simulink model "Cascaded_LQR"  (R2021a)
settings: Solver=VariableStepAuto  StartTime=0.0  StopTime=inf  RelTol=1e-3
values from neighbouring files (symbols this model uses):
  dragCoeffMov = 0.01    [param_set.m]
  g = 9.8    [param_set.m]
  m = 1.5    [param_set.m]
  set_points = [1 0 hover_height 0 0 0 0 0 0 0 0 0]'    [linearize_lqr.m]    (also in param_set.m)
  u_eq = [T_eq 0 0 0]    [linearize_lqr.m]    (also in param_set.m = [-m*g 0 0 0])
  windVel = [0 0 0]'    [param_set.m]
undefined symbols (not defined in the file or in its folder): lqr_K
libraries: shared6dof x1, sharedtransform x1, uavutilslib x1
settings Model: Creator=willwu  LastModifiedBy=willwu

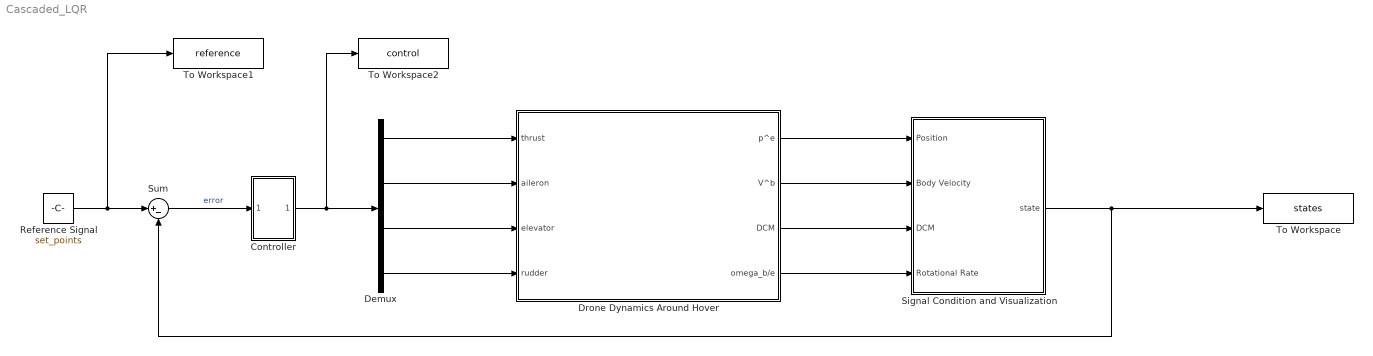
== system Cascaded_LQR ==
  Controller : Subsystem
  Demux : Demux
  Drone Dynamics Around Hover : Subsystem
  Reference Signal : Constant  Value=set_points
  Signal Condition and Visualization : Subsystem
  Sum : Sum  Inputs=|+-
  To Workspace : ToWorkspace  VariableName=states  SaveFormat=Structure With Time  SampleTime=-1
  To Workspace1 : ToWorkspace  VariableName=reference  SaveFormat=Structure With Time  SampleTime=-1
  To Workspace2 : ToWorkspace  VariableName=control  SaveFormat=Structure With Time  SampleTime=-1
  wires:
  Demux/1 -> Drone Dynamics Around Hover/1(thrust)
  Demux/2 -> Drone Dynamics Around Hover/2(aileron)
  Demux/3 -> Drone Dynamics Around Hover/3(elevator)
  Demux/4 -> Drone Dynamics Around Hover/4(rudder)
  Reference Signal/1 -> To Workspace1/1, Sum/1
  Sum/1 -> Controller/1(In1)  "error"
  Controller/1(Out1) -> Demux/1, To Workspace2/1
  Signal Condition and Visualization/1(state) -> Sum/2, To Workspace/1
  Drone Dynamics Around Hover/1(p^e) -> Signal Condition and Visualization/1(Position)
  Drone Dynamics Around Hover/2(V^b) -> Signal Condition and Visualization/2(Body Velocity)
  Drone Dynamics Around Hover/3(DCM) -> Signal Condition and Visualization/3(DCM)
  Drone Dynamics Around Hover/4(omega_b/e) -> Signal Condition and Visualization/4(Rotational Rate)

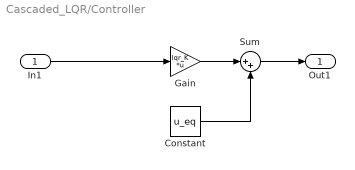
== system Cascaded_LQR/Controller ==
  In1 : Inport
  Constant : Constant  Value=u_eq
  Gain : Gain  Gain=lqr_K  Multiplication=Matrix(K*u)
  Sum : Sum  Inputs=|++
  Out1 : Outport
  wires:
  In1/1 -> Gain/1
  Gain/1 -> Sum/1
  Sum/1 -> Out1/1
  Constant/1 -> Sum/2

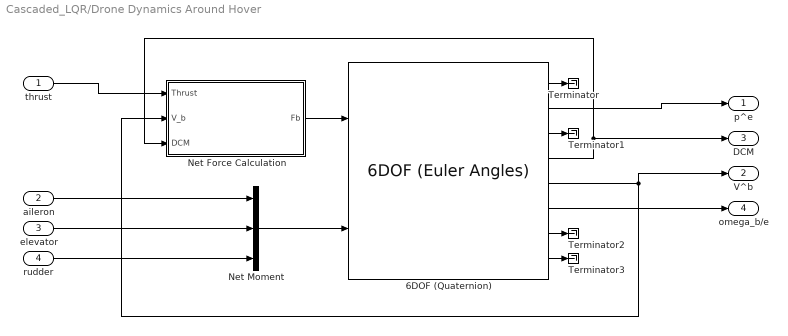
== system Cascaded_LQR/Drone Dynamics Around Hover ==
  thrust : Inport
  aileron : Inport  Port=2
  elevator : Inport  Port=3
  rudder : Inport  Port=4
  6DOF (Quaternion) : shared6dof/6DOF (Euler Angles)  units=Metric (MKS)  mtype=Fixed  rep=Quaternion  xme_0=[0 0 0]  Vm_0=[0 0 0]  eul_0=[0 0 0]  pm_0=[0 0 0]  mass_0=m  mass_e=0.5  mass_f=2.0  inertia=J  inertia_e=eye(3)  inertia_f=2*eye(3)  k_quat=1.0  vre_flag=on  abi_flag=off  aMode=0  xme_statename=''  Vm_statename=''  eul_statename=''  quat_statename=''  pm_statename=''  mass_statename=''
      settings: SourceProductBaseCode=AE,PW,DR,MT,UV,VE
  Net Force Calculation : Subsystem
  Net Moment : Mux  Inputs=3
  Terminator{,1..3} (4 alike) : Terminator
  p^e : Outport
  V^b : Outport  Port=2
  DCM : Outport  Port=3
  omega_b/e : Outport  Port=4
  wires:
  aileron/1 -> Net Moment/1
  rudder/1 -> Net Moment/3
  Net Moment/1 -> 6DOF (Quaternion)/2
  6DOF (Quaternion)/5 -> V^b/1, Net Force Calculation/2(V_b)
  6DOF (Quaternion)/6 -> omega_b/e/1
  6DOF (Quaternion)/4 -> DCM/1, Net Force Calculation/3(DCM)
  6DOF (Quaternion)/2 -> p^e/1
  thrust/1 -> Net Force Calculation/1(Thrust)
  Net Force Calculation/1(Fb) -> 6DOF (Quaternion)/1
  elevator/1 -> Net Moment/2
  6DOF (Quaternion)/1 -> Terminator/1
  6DOF (Quaternion)/3 -> Terminator1/1
  6DOF (Quaternion)/7 -> Terminator2/1
  6DOF (Quaternion)/8 -> Terminator3/1

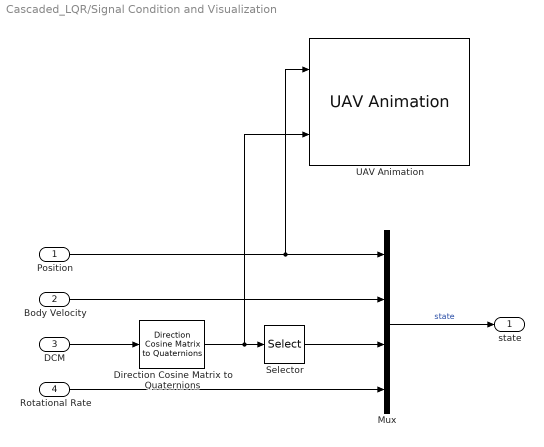
== system Cascaded_LQR/Signal Condition and Visualization ==
  Position : Inport
  Body Velocity : Inport  Port=2
  DCM : Inport  Port=3
  Rotational Rate : Inport  Port=4
  Direction Cosine Matrix to Quaternions : sharedtransform/Direction Cosine Matrix  to Quaternions  aMode=0  action=None  tolerance=eps(2)
      settings: SourceProductBaseCode=AE,PW,DR,MT,UV,VE
  Mux : Mux
  Selector : Selector  InputPortWidth=4  IndexOptions=Index vector (dialog)  Indices=[2 3 4]  OutputSizes=1
  UAV Animation : uavutilslib/UAV Animation  UAVType=Multirotor  UAVSize=1  InertialZDirection=Down  SampleTime=-1
      settings: SourceProductBaseCode=UV
  state : Outport
  wires:
  Selector/1 -> Mux/3
  Position/1 -> Mux/1, UAV Animation/1
  Body Velocity/1 -> Mux/2
  Rotational Rate/1 -> Mux/4
  Mux/1 -> state/1  "state"
  DCM/1 -> Direction Cosine Matrix to Quaternions/1
  Direction Cosine Matrix to Quaternions/1 -> Selector/1, UAV Animation/2

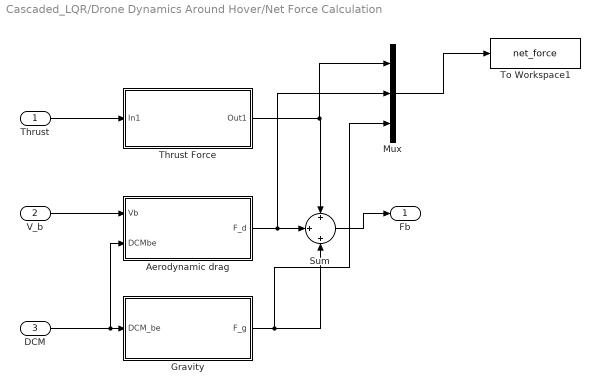
== system Cascaded_LQR/Drone Dynamics Around Hover/Net Force Calculation ==
  Thrust : Inport
  V_b : Inport  Port=2
  DCM : Inport  Port=3
  Aerodynamic drag : Subsystem
  Gravity : Subsystem
  Mux : Mux  Inputs=3
  Sum : Sum  Inputs=+|+|+
  Thrust Force : Subsystem
  To Workspace1 : ToWorkspace  VariableName=net_force  SaveFormat=Structure With Time  SampleTime=-1
  Fb : Outport
  wires:
  DCM/1 -> Aerodynamic drag/2(DCMbe), Gravity/1(DCM_be)
  Gravity/1(F_g) -> Mux/3, Sum/3
  Sum/1 -> Fb/1
  Thrust/1 -> Thrust Force/1(In1)
  Thrust Force/1(Out1) -> Mux/1, Sum/1
  V_b/1 -> Aerodynamic drag/1(Vb)
  Aerodynamic drag/1(F_d) -> Mux/2, Sum/2
  Mux/1 -> To Workspace1/1

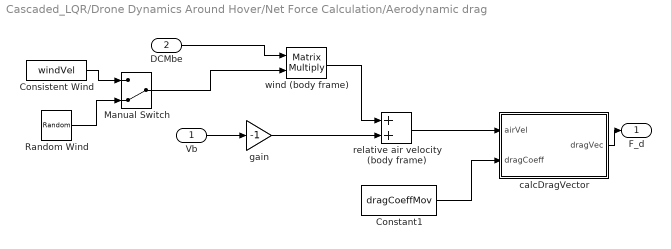
== system Cascaded_LQR/Drone Dynamics Around Hover/Net Force Calculation/Aerodynamic drag ==
  Vb : Inport
  DCMbe : Inport  Port=2
  Consistent Wind : Constant  Value=windVel
  Constant1 : Constant  Value=dragCoeffMov
  Manual Switch : ManualSwitch  CurrentSetting=0
  Random Wind : RandomNumber  Mean=[0 1.5 1.3]'  Variance=[2 2 1]'  SampleTime=0.1  VectorParams1D=off
  calcDragVector : MATLAB Function  TreatAsAtomicUnit=on
  gain : Gain  Gain=-1
  relative air velocity (body frame) : Sum
  wind (body frame) : Product  Multiplication=Matrix(*)
  F_d : Outport
  wires:
  Vb/1 -> gain/1
  calcDragVector/1(dragVec) -> F_d/1
  relative air velocity (body frame)/1 -> calcDragVector/1(airVel)
  gain/1 -> relative air velocity (body frame)/2
  Constant1/1 -> calcDragVector/2(dragCoeff)
  DCMbe/1 -> wind (body frame)/1
  wind (body frame)/1 -> relative air velocity (body frame)/1
  Consistent Wind/1 -> Manual Switch/1
  Random Wind/1 -> Manual Switch/2
  Manual Switch/1 -> wind (body frame)/2

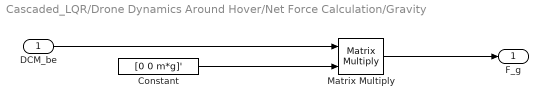
== system Cascaded_LQR/Drone Dynamics Around Hover/Net Force Calculation/Gravity ==
  DCM_be : Inport
  Constant : Constant  Value=[0 0 m*g]'
  Matrix Multiply : Product  Multiplication=Matrix(*)
  F_g : Outport
  wires:
  Constant/1 -> Matrix Multiply/2
  DCM_be/1 -> Matrix Multiply/1
  Matrix Multiply/1 -> F_g/1

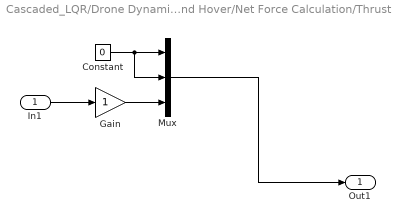
== system Cascaded_LQR/Drone Dynamics Around Hover/Net Force Calculation/Thrust Force ==
  In1 : Inport
  Constant : Constant  Value=0
  Gain : Gain
  Mux : Mux  Inputs=3
  Out1 : Outport
  wires:
  Constant/1 -> Mux/2, Mux/1
  In1/1 -> Gain/1
  Mux/1 -> Out1/1
  Gain/1 -> Mux/3

== matlab function Cascaded_LQR/Drone Dynamics Around Hover/Net Force Calculation/Aerodynamic drag/calcDragVector ==
  data: airVel input; dragVec output; dragCoeff input
function dragVec = fcn(airVel, dragCoeff)

dragVec = dragCoeff * norm(airVel) * airVel;

end
